simulink model "Final_Model_Building_2_AirflowAdded"  (R2022a)
settings: Solver=ode1  StartTime=0.0  StopTime=24*3600  FixedStep=10  RelTol=1e-3
values from neighbouring files (symbols this model uses):
  Aux_Threshold = 52    [Setup_Code_EWASP_VC.m]
  buildingAge = 2005    [Setup_Code_EWASP_VC.m]
  ceilingHeight = 2.4    [Setup_Code_EWASP_VC.m]
  conductiveHconnectMatrix = [ ... (first row only)    [Setup_Code_EWASP_VC.m]
  cRoofGreen = 100000    [Setup_Code_EWASP_VC.m]
  Defrost_After_Time = 30    [Setup_Code_EWASP_VC.m]
  DHWDemandProfile = occFreegainHotwaterElecTestPassiveOcc3(:,3)    [Setup_Code_EWASP_VC.m]
  Elec_Max = Elec_Max*(30/24.2)    [Setup_Code_EWASP_VC.m]
  Elec_Mid = Elec_Mid*(30/24.2)    [Setup_Code_EWASP_VC.m]
  Elec_Min = Elec_Min*(30/24.2)    [Setup_Code_EWASP_VC.m]
  ElecDemandProfile = occFreegainHotwaterElecTestPassiveOcc3(:,4)    [Setup_Code_EWASP_VC.m]
  ElecFixed = [Elec_Max(6,2) Elec_Max(6,4) Elec_Max(6,6) Elec_Max(6,7) ... (first row only)    [Setup_Code_EWASP_VC.m]
  floorOrCeilingArea = floorOrCeilingArea*1.15    [Setup_Code_EWASP_VC.m]
  forceCold = 0    [Setup_Code_EWASP_VC.m]
  freegain = occFreegainHotwaterElecTestPassiveOcc3(:,2)-max(occupancy)*25    [Setup_Code_EWASP_VC.m]
  furnitureModelOn = 1    [Setup_Code_EWASP_VC.m]
  Heat_Max = Heat_Max*(30/24.2)    [Setup_Code_EWASP_VC.m]
  Heat_Mid = Heat_Mid*(30/24.2)    [Setup_Code_EWASP_VC.m]
  Heat_Min = Heat_Min*(30/24.2)    [Setup_Code_EWASP_VC.m]
  HeatFixed = [Heat_Max(6,2) Heat_Max(6,4) Heat_Max(6,6) Heat_Max(6,7) ... (first row only)    [Setup_Code_EWASP_VC.m]
  HeatingOnProfile = repmat(HeatingOnProfile,365,1)    [Setup_Code_EWASP_VC.m]
  HEX_ReturnLowerLimit = 52.5    [Setup_Code_EWASP_VC.m]
  HEX_ReturnUpperLimit = 55    [Setup_Code_EWASP_VC.m]
  LeakMultiplier = 1+(2*(rand()-0.5)/10)    [Setup_Code_EWASP_VC.m]
  maxOcc = max(occupancyProfile)    [Setup_Code_EWASP_VC.m]
  NESW_wallArea = max(NESW_Lengths*ceilingHeight-NESW_Windows,0)    [Setup_Code_EWASP_VC.m]
  NESW_Windows = [ ... (first row only)    [Setup_Code_EWASP_VC.m]
  numRooms = roomCount    [Setup_Code_EWASP_VC.m]
  occupancy = occupancyProfile    [Setup_Code_EWASP_VC.m]
  offsetDays = 0    [Setup_Code_EWASP_VC.m]
  pumpChoice = pumpChoices(MinIndex,1)    [Setup_Code_EWASP_VC.m]
  pumpRamp = 180    [Setup_Code_EWASP_VC.m]
  ReturnLowerLimit = 37.5    [Setup_Code_EWASP_VC.m]
  ReturnUpperLimit = 40    [Setup_Code_EWASP_VC.m]
  RoofIrradiance = Flat_NS_EW_RoofIrradiance(:,1)    [Setup_Code_EWASP_VC.m]
  roofStartTemp = ones(11,1)*20    [Setup_Code_EWASP_VC.m]
  rooftype = 0    [Setup_Code_EWASP_VC.m]
  RoomDataMatrix = [zeros(1,12);ones(1,12)*wallDensity;zeros(1,12);ones(1,12)*wallU;ones(1,12)*windowU;ones(1,12)*floorU;ones(1,12)*ceilingU;zeros(1,12);windowArea, 0;floorOrCeilingArea;zeros(1,12);floorOrCeilingArea*ceilingHeight]    [Setup_Code_EWASP_VC.m]
  roomVol = roomVol*1.15    [Setup_Code_EWASP_VC.m]
  slabStartTemp = (GroundTempTimeSeries(offsetDays*1440+1,1)+thermostatSetting)/2    [Setup_Code_EWASP_VC.m]
  SlackRequest = zeros(1440,1)    [Setup_Code_EWASP_VC.m]
  SolarThermalExists = 0    [Setup_Code_EWASP_VC.m]
  SourceFixed = HeatFixed-ElecFixed    [Setup_Code_EWASP_VC.m]
  StateSeries = StateSeriesGenerator(22,7,1)    [Setup_Code_EWASP_VC.m]
  Tank_Lower_Temp = 49.5    [Setup_Code_EWASP_VC.m]
  Tank_Upper_Temp = 52    [Setup_Code_EWASP_VC.m]
  Tank_Volume_m3 = 0.15    [Setup_Code_EWASP_VC.m]
  TankHeatHour = randi([1 5])-1    [Setup_Code_EWASP_VC.m]
  upDown = [0;0;0;0;1;1;1;1;1;1;1]    [Setup_Code_EWASP_VC.m]
  wallStartTempExt = thermostatSetting*(0.266+0.00215*outdoorStartTemp+0.018*wallU+0.00113*outdoorStartTemp*wallU+0.0068*wallU^2)    [Setup_Code_EWASP_VC.m]
undefined symbols (not defined in the file or in its folder): a, ceilingU, condUDMatrix, convUDMatrix, deltaPEXPANDED_E, deltaPEXPANDED_E2, deltaPEXPANDED_N, deltaPEXPANDED_N2, deltaPEXPANDED_S, deltaPEXPANDED_S2, deltaPEXPANDED_W, deltaPEXPANDED_W2, DesiredDHWTemp, DesiredFlowTempVsInOutDeltaTemp, DiffuseHorizontal, DiscIntNeverNeededParam, DNI, dwnAndConcrete, DWORK_A_HX, DWORK_CHK_FLU, DWORK_CP_NODE, DWORK_DH, DWORK_FLUID, DWORK_HCON, DWORK_LOSS, DWORK_MDOTDOWN, DWORK_MDOTIN, DWORK_MDOTUP, DWORK_MIX, DWORK_PRESS, DWORK_QDOTIN, DWORK_RHO_NODE, DWORK_TIN, DWORK_TS_OLD, DWORK_V_NODE, ExtractRates, GroundTempTimeSeries, HCM, HCM2, HCM_closed, HCM_closed2, intermediateU, IsTop, massFlowMatrix, mechEfficiency, neighbourMatrix, numericalRoomUse, RadiatorMatrix, room2roomflowmatrix_E, room2roomflowmatrix_E2, room2roomflowmatrix_N, room2roomflowmatrix_N2, room2roomflowmatrix_S, room2roomflowmatrix_S2, room2roomflowmatrix_W, room2roomflowmatrix_W2, StateAirInEXPANDED_E, StateAirInEXPANDED_E2, StateAirInEXPANDED_N, StateAirInEXPANDED_N2 ... (+27)
libraries: simulink x6, dspsigops x4, dspmtrx3 x4, carnot x3, spsEdgeDetectorLib x2, dspstat3 x2, powerlib_meascontrol x1, simulink_extras x1
(part 6 of 27)

== system Final_Model_Building_2_AirflowAdded/GSHP_Subsystem/DHW for GSHP case ==
  note: immediately adds value to integrator to ensure legionella cycle doesnt begin right away (allows different start times)
  note: reset integrator at 00:00+delay every day,
      | so legionella cycle can start agin
  note: Makes the tank heat up to 60oC only once - only starts when the threshold programmed into switch A is hit
  note: this part prevents heating
      | to 60oC more than once per
      | day
  In1 : Inport
  In2 : Inport  Port=2
  In3 : Inport  Port=3
  In4 : Inport  Port=4
  In5 : Inport  Port=5
  In6 : Inport  Port=6
  1 means loop has been running for less than 15 mins : Switch  Criteria=u2 > Threshold  Threshold=900  SaturateOnIntegerOverflow=off  InputSameDT=off
  "1 means pump is on, and therefore ground loop is on" : Switch  Criteria=u2 > Threshold  Threshold=0.5  SaturateOnIntegerOverflow=off  InputSameDT=off
  1 means return temp recently fell below 52.1 : Relay  OnSwitchValue=61  OffSwitchValue=59  OnOutputValue=0  OffOutputValue=1  OutDataTypeStr=boolean
  1 means return temp recently fell below 52.5 : Relay  OnSwitchValue=55  OffSwitchValue=52.5  OnOutputValue=0  OffOutputValue=1  OutDataTypeStr=boolean
  1-D Lookup Table : Lookup_n-D  Commented=on  NumberOfTableDimensions=1  BreakpointsForDimension1=[0:100]  Table="[1  1\t1\t1\t1\t1\t1\t1\t1\t1\t1\t1\t1\t1\t1\t1\t1\t1\t1\t1\t1\t1\t1\t1\t1\t1\t1\t1\t1\t1\t1\t1\t1\t1\t1\t1\t1\t1\t1\t1\t1\t1\t1\t0.964285714285714\t0.931034482758621\t0.900000000000000\t0.870967741935484\t0.843750000000000\t0.818181818181818\t0.794117647058824\t0.771428571428572\t0.750000000000000\t0.729729729729730\t0.710526315789474\t0.692307692307692\t0.675000000000000\t0.658536585365854\t0.642857142857143\t0.627906976744186\t0.613636363636364\t0.600000000000000\t0.586956521739130\t0.574468085106383\t0.562500000000000\t0.551020408163265\t0.540000000000000\t0.529411764705882\t0.519230769230769\t0.509433962264151\t0.500000000000000\t0.490909090909091\t0.482142857142857\t0.473684210526316\t0.465517241379310\t0.457627118644068\t0.450000000000000\t0.442622950819672\t0.435483870967742\t0.428571428571429\t0.421875000000000\t0.415384615384615\t0.409090909090909\t0.402985074626866\t0.397058823529412\t0.391304347826087\t0.385714285714286\t0.380281690140845\t0.375000000000000\t0.369863013698630\t0.364864864864865\t0.360000000000000\t0.355263157894737\t0.350649350649351\t0.346153846153846\t0.341772151898734\t0.337500000000000\t0.333333333333333\t0.329268292682927\t0.325301204819277\t0.321428571428571\t0.317647058823529]"  InternalRulePriority=Speed  RndMeth=Simplest
  Aux Heater on1 : Logic  Inputs=3  AllPortsSameDT=off  OutDataTypeStr=boolean
  Bus Selector1 : BusSelector  OutputSignals=Pelec  OutputAsBus=on
  C/C++ Code Block : S-Function  InitFcn=try, set_param(gcb,'FunctionName','Select_sensor_mid'), end  FunctionName=Select_sensor_mid  SFunctionModules=Select_sensor_mid_wrapper  SFunctionDeploymentMode=off  EnableBusSupport=off  mask(S-Function Builder){}
      mask help: Simulink:masks:SFunctionBuilder_MD
      mask init: same as Final_Model_Building_2_AirflowAdded/ASHP_Subsystem/DHW for ASHP Case/C/C++ Code Block
      settings: CopyFcn=set_param(gcbh,'LinkStatus','none')  PreSaveFcn=try, set_param(gcb,'FunctionName','Select_sensor_mid'), end  OpenFcn=sfunctionwizard(gcbh)
      mask Display: plot(val(:,1),val(:,2)),disp(sys), port_label('input',1,'u0'), port_label('output',1,'y0')
  CHANGE to prevent 60oC being hit too often : Switch  Threshold=1  SaturateOnIntegerOverflow=off  InputSameDT=off
  Cast To Double : DataTypeConversion  OutDataTypeStr=double  SaturateOnIntegerOverflow=off  RndMeth=Floor
  Cast To Double2 : DataTypeConversion  OutDataTypeStr=double  SaturateOnIntegerOverflow=off  RndMeth=Floor
  Cast To Double3 : DataTypeConversion  OutDataTypeStr=double  SaturateOnIntegerOverflow=off  RndMeth=Floor
  Constant{1,5..6,10} (4 alike) : Constant  Value=0
  Constant11 : Constant
  Constant12 : Constant  Value=0.333
  Constant2 : Constant  Value=0.1
  Constant3 : Constant  Value=24*3600
  Constant4 : Constant
  Constant7 : Constant  Value=12
  Constant8 : Constant
  Constant9 : Constant  Value=DesiredDHWTemp
  Delay : Delay  DelayLength=1  InitialCondition=0
  Delay1 : Delay  DelayLength=1  InitialCondition=0
  Delay2 : Delay  DelayLength=1+TankHeatHour*(3600/5)  InitialCondition=0
  Delay4 : Delay  DelayLength=1  InitialCondition=0
  Digital Clock1 : DigitalClock  SampleTime=10
  Digital Clock2 : DigitalClock  SampleTime=10
  Discrete-Time Integrator : DiscreteIntegrator  ExternalReset=rising  SampleTime=-1  OutDataTypeStr=double  ICPrevOutput=DiscIntNeverNeededParam  ICPrevScaledInput=DiscIntNeverNeededParam
  Divide : Product  Inputs=*/
  Edge Detector : powerlib_meascontrol/Logic/Edge Detector  model=Rising  ic=0  Ts=-1
      settings: SourceProductBaseCode=PS
  HeatPump_Simplified : Subsystem  AncestorBlock=carnot/Source/Heat_Pump/HeatPump  mask(heat pump){Tcin=[-5 7 12], Thout=[35 45 55 60], Qdotc=[4400*a-2000*a 4200*a-2000*a 3200*a-2000*a 1800*a-2000*a;5800*a-2100*a 5500*a-2100*a 4200*a-2100*a 2800*a-2100*a;8400*a-2200*a 7200*a-2200*a 5500*a-2200*a 3300*a-2200*a], Qdoth=[4400*a 4200*a 3200*a 1800*a;5600*a 5500*a 4200*a 2800*a;8400*a 7200*a 5500*a 3300*a], Pel=[2000*a 2000*a 2000*a 2000*a;2100*a 2100*a 2100*a 2100*a;2200*a 2200*a 2200*a 2200*a], caph=10*4180, capc=4180*225, UA=7, linc=10, quac=10, linh=10, quah=10}
      mask prompts: Tcin "inlet source temperature vector (°C)"; Thout "outlet load temperature vector (°C)"; Qdotc "source power matrix (W)"; Qdoth "heating power matrix (W)"; Pel "electric power matrix (W)"; caph "thermal capacity hot loop [J/K]"; capc "thermal capacity cold loop [J/K]"; UA "heat loss coefficient [W/K]"; linc "Cold side linear massflow dependant pressure drop in [Pa*s/kg]"; quac "Cold side quadratic massflow dependant pressure drop hot side in [Pa*s²/kg]"; linh "Hot side linear massflow dependant pressure drop in [Pa*s/kg]"; quah "Hot side quadratic massflow dependant pressure drop hot side in [Pa*s²/kg]"
      mask help:
      | Linearized heat pump model. Uses measured data according to EN 14511 as input.
      | heating power: Qdot_h = K1*Tcold_in + K2*Thot_out + K3
      | electric power: Pel = K4*Tcold_in + K5*Thot_out + K6
      | source power: Qdot_c = -K7*Tcold_in - K8*Thot_out - K9
      | differential equation: cap*dTh/dt = Qdot + mdot*cp*(T_in-T) + UA*(Tamb-T)
      | with: cap = mass * heat_capactiy
      | See hp_param.m for the parameters K1 to K9.
      | Literature: Schwamberger, K.: Fortschrittsberichete VDI, Nr. 263, 1991
      mask init: same as Final_Model_Building_2_AirflowAdded/ASHP_Subsystem/DHW for ASHP Case/HeatPump_Simplified1
      mask Help: web(fullfile(path_carnot('help'),'heatpump.html'),'-helpbrowser')
      mask DialogControl ParameterTabVar0 Prompt: HP Caracteristic
      mask DialogControl ParameterTabVar01 Prompt: Thermal
      mask DialogControl ParameterTabVar012 Prompt: Hydraulic
      mask Display: plot(-20,-10,120,110,[10,20,40,60,80,90,90,80,60,40,20,10,10],[60,80,90,90,80,60,40,20,10,10,20,40,60],[40,20],[90,20],[60,80],[90,20],[50,50],[30,50],[60,40],[40,40],[57,43],[33,46],[44,57],[34,46])
  Ii : Logic  AllPortsSameDT=off  OutDataTypeStr=boolean
  Logical Operator : Logic  AllPortsSameDT=off  OutDataTypeStr=boolean
  Massflow when system is off1 : Constant  Value=0
  Max of Elements : MinMax  Function=max  Inputs=2
  Minus : Sum  Inputs=+-
  Minus1 : Sum  Inputs=+-
  Minus2 : Sum  Inputs=2
  Mod1 : Math  Operator=mod  SignedPower=on
  No DHW operation from Heat Pump : Constant  Value=0
  Plus : Sum
  Plus1 : Sum
  Product : Product
  "Run loop if either - heaing system is on, heating system was activated less than 15 mins ago" : Logic  Operator=OR  AllPortsSameDT=off  OutDataTypeStr=boolean
  S-Function Builder : S-Function  InitFcn=try, set_param(gcb,'FunctionName','Select_sensor'), end  FunctionName=Select_sensor  SFunctionModules=Select_sensor_wrapper  SFunctionDeploymentMode=off  EnableBusSupport=off  mask(S-Function Builder){}
      mask help: Simulink:masks:SFunctionBuilder_MD
      mask init: same as Final_Model_Building_2_AirflowAdded/ASHP_Subsystem/DHW for ASHP Case/C/C++ Code Block
      settings: CopyFcn=set_param(gcbh,'LinkStatus','none')  PreSaveFcn=try, set_param(gcb,'FunctionName','Select_sensor'), end  OpenFcn=sfunctionwizard(gcbh)
      mask Display: plot(val(:,1),val(:,2)),disp(sys), port_label('input',1,'u0'), port_label('output',1,'y0')
  SWITCH A : Switch  Threshold=Aux_Threshold  SaturateOnIntegerOverflow=off  InputSameDT=off
  Saturation : Saturate  UpperLimit=1  LowerLimit=0
  Scope{,1..12} (13 alike) : Scope
  Storage_Type_2_CONF : Subsystem  AncestorBlock=carnot/Storage/Thermal/Storage_Type_2_CONF  mask(Storage for hot water production){t0=52.1, hgt=1.5279, stgtype=2, tini=[52.1 52.1 52.1 52.1 52.1 52.1 52.1 52.1 52.1 52.1], mpts=[1 2 3 4 5 6 7 8 9 10], PathName=fullfile(pwd,'TankVolTemp'), FileName='<user defined>', userPath=on, userParam=on, uwall=0.235, ubot=0.235, utop=0.235, axcond=0.235, volume=Tank_Volume_m3, dia=((4/(3*3.142))*Tank_Volume_m3)^(1/3), standing=standing cylinder, nodes=10, mpoints=10, Tsensor=[0.1:0.1:0.9], hx1inlet=0.45, hx1outlet=0, hx1dia=0.03, hx1uac=500, hx1uam=0.15, hx1uat=0.6, hx1dpqua=20, hx1dplin=20, pipe1inlet=0, pipe1outlet=1, pipe1dia=0.03, pipe2inlet=0.6, pipe2outlet=1, pipe2dia=0.03}
      mask prompts: t0 "Initial temperature (vector or scalar) in °C"; hgt "Height of storage in m"; stgtype "Storage Type (0..5)"; tini "Start temperatures of nodes in °C"; mpts "Index to measured nodes"; PathName "Path"; FileName "Parameter set"; userPath "Edit path and name of parameter set"; userParam "User defined parameters"; uwall "Heat transfer coefficient to ambient [W/m²K]"; ubot "Heat transfer coefficient to ambient bottom [W/m²K]"; utop "Heat transfer coefficient to ambient top [W/m²K]"; axcond "Effective thermal conductivity [W/m/K]"; volume "Volume [m³]"; dia "Diameter [m]"; standing "Position"; nodes "Number of nodes"; mpoints "Number of node temperatures (for display)"; Tsensor "Temperature sensor position (0..1, 0 = bottom, 1 = top)"; hx1inlet "relative height of inlet"; hx1outlet "relative height of outlet"; hx1dia "Diameter of HX pipe [m]"; hx1uac "uac: heat transfer coefficient [W/K /(kg/s) /(°C)]"; hx1uam "uam: massflow dependent heat transfer [-]"; hx1uat "uat: temperature difference dependent heat transfer [-]"; hx1dpqua "pressure drop quadratic in mdot [Pa*s²/kg²]"; hx1dplin "pressure drop linear in mdot [Pa*s/kg]"; pipe1inlet "relative height of inlet, range from 0 (= bottom) to 1 (= top)"; pipe1outlet "relative height of outlet, range from 0 (= bottom) to 1 (= top)"; pipe1dia "Diameter of pipe in m"; pipe2inlet "relative height of inlet, range from 0 (= bottom) to 1 (= top)"; pipe2outlet "relative height of outlet, range from 0 (= bottom) to 1 (= top)"; pipe2dia "Diameter of pipe in m"
      mask help:
      | Storage for hot water production (domestic hot water cylinder). The storage model has the following components (with their typical position):
      | - one charging heat exchanger (lower part)
      | - one pipe connection for the hot water (total height)
      | - one pipe connection for the hot water circulation (upper part )
      mask init:
      | %[ok, param] = CarnotCallbacks_StorageConf('SetParam',stgtype,gcbh,PathName,FileName);
      mask Help: web(fullfile(path_carnot('help'),'Storage_Type_N.html'),'-helpbrowser')
      mask TypeOptions hgt: HX_EN12977_1/hgt | Pipe_Connection_1/hgt | Pipe_Connection_2/hgt
      mask TypeOptions stgtype: CreateSdat/stgtype
      mask TypeOptions tini: sfun_storageTnodesjh/tini
      mask TypeOptions mpts: select_T/Indices
      mask Callback userPath: [ok, param] = CarnotCallbacks_StorageConf('UserEdit',2,gcbh);
      mask Callback userParam: [ok, param] = CarnotCallbacks_StorageConf('UserEdit',2,gcbh);
      mask TypeOptions uwall: sfun_storageTnodesjh/uloss
      mask TypeOptions ubot: sfun_storageTnodesjh/ubot
      mask TypeOptions utop: sfun_storageTnodesjh/utop
      mask TypeOptions axcond: sfun_storageTnodesjh/cond
      mask TypeOptions volume: sfun_storageTnodesjh/volume
      mask TypeOptions dia: sfun_storageTnodesjh/dia
      mask TypeOptions standing: sfun_storageTnodesjh/standing
      mask TypeOptions nodes: sfun_storageTnodesjh/nodes | select_T/InputPortWidth | HX_EN12977_1/nodes | HX_EN12977_2/nodes | HX_EN12977_3/nodes | Pipe_Connection_1/nodes | Pipe_Connection_2/nodes | Pipe_Connection_3/nodes
      mask TypeOptions Tsensor: T_Sensor_Surface/pos
      mask TypeOptions hx1inlet: HX_EN12977_1/h_in
      mask TypeOptions hx1outlet: HX_EN12977_1/h_out
      mask TypeOptions hx1dia: HX_EN12977_1/dia
      mask TypeOptions hx1uac: HX_EN12977_1/ua0
      mask TypeOptions hx1uam: HX_EN12977_1/uam
      mask TypeOptions hx1uat: HX_EN12977_1/uat
      mask TypeOptions hx1dpqua: HX_EN12977_1/dpqua
      mask TypeOptions hx1dplin: HX_EN12977_1/dplin
      mask TypeOptions pipe1inlet: Pipe_Connection_1/h_in
      mask TypeOptions pipe1outlet: Pipe_Connection_1/h_out
      mask TypeOptions pipe1dia: Pipe_Connection_1/dia
      mask TypeOptions pipe2inlet: Pipe_Connection_2/h_in
      mask TypeOptions pipe2outlet: Pipe_Connection_2/h_out
      mask TypeOptions pipe2dia: Pipe_Connection_2/dia
      mask DialogControl Container14 Prompt: Infos
      mask DialogControl ParameterGroupVar Prompt: Picking a parameter set
      mask DialogControl Control3 Prompt: Carnot public data
      mask DialogControl Control3 Callback: [ok, file] = CarnotCallbacks_StorageConf('GetFilename',2,gcbh,'public');
      mask DialogControl Control4 Prompt: Carnot internal data
      mask DialogControl Control4 Callback: [ok, file] = CarnotCallbacks_StorageConf('GetFilename',2,gcbh,'internal');
      mask DialogControl Control2 Prompt: Selected path
      mask DialogControl Control2 Callback: [ok, file] = CarnotCallbacks_StorageConf('GetFilename',2,gcbh,'selected');
      mask DialogControl Container4 Prompt: Parameter values
      mask DialogControl Container6 Prompt: Storage
      mask DialogControl Container8 Prompt: Connections
      mask DialogControl Container11 Prompt: Heat exchanger
      mask DialogControl Container9 Prompt: Discharging pipe
      mask DialogControl Container12 Prompt: Circulation pipe
      mask DialogControl Control6 Prompt: Save in Carnot internal data
      mask DialogControl Control6 Callback: [ok, param] = CarnotCallbacks_StorageConf('SaveFilename',2,gcbh,'internal','STG');
      mask DialogControl Control5 Prompt: Save in selected path
      mask DialogControl Control5 Callback: [ok, param] = CarnotCallbacks_StorageConf('SaveFilename',2,gcbh,'selected','STG');
      mask Display:
      | % user defined picture file
      | namestr = ['Storage_Type_', num2str(get_param(gcb,'stgtype'))];
      | picfile = fullfile(path_carnot('intlibsl'), 'Storage','Thermal', ...
      |     namestr,'parameter_set', [namestr, '.jpg']);
      | 
      | % show public picture
      | plot([36,36,40,50,54,54,50,40,36]/90,...
      |     [90,50,45,45,50,90,93,93,90]/100,[36,51,44,51,36]/90,...
      |     [50,50,55,60,60]/100)
      | set_param(gcb, 'BackgroundColor', 'Red')
      | 
      | % show internal picture if defined
      | if  ~BlockIsInCarnotLibrary       % if not located in library
      |     if exist(picfile, 'file')
      |         image(imread(picfile), [0.25, 0, 0.45, 1])
      |         set_param(gcb, 'BackgroundColor', 'White')
      |     end
      | end
  Subsystem : Subsystem
      mask Display:
      | disp('Minute to \n Second Res')
      | port_label('input', 1, 'min res')
      | port_label('output', 1, 'sec res')
  Sum4 : Sum  Inputs=|++
  Switch : Switch  Criteria=u2 > Threshold  Threshold=0.1  SaturateOnIntegerOverflow=off  InputSameDT=off
  Switch Case : SwitchCase  CaseConditions={1,0}
  Switch Case Action Subsystem : Subsystem  TreatAsAtomicUnit=on
  Switch Case Action Subsystem1 : Subsystem  TreatAsAtomicUnit=on
  Switch Case Action Subsystem2 : Subsystem  TreatAsAtomicUnit=on
  Switch Case Action Subsystem3 : Subsystem  TreatAsAtomicUnit=on
  Switch Case1 : SwitchCase  CaseConditions={1,0}
  Switch1 : Switch  Criteria=u2 > Threshold  Threshold=0.5  SaturateOnIntegerOverflow=off  InputSameDT=off
  Switch5 : Switch  Criteria=u2 > Threshold  Threshold=0.5  SaturateOnIntegerOverflow=off  InputSameDT=off
  Tank Exists : Constant  Value=tankExists
  Terminator : Terminator
  Terminator1 : Terminator
  Terminator2 : Terminator
  Time since loop started flowing : Integrator  ExternalReset=rising
  over1 : Switch  Threshold=60  SaturateOnIntegerOverflow=off  InputSameDT=off
  over2 : Switch  Criteria=u2 > Threshold  SaturateOnIntegerOverflow=off  InputSameDT=off
  z{1,4,6,9} (4 alike) : Constant  Value=0
  z{2,5,7..8} (4 alike) : Constant
  Out1 : Outport  VectorParamsAs1DForOutWhenUnconnected=off
  Out2 : Outport  Port=2  VectorParamsAs1DForOutWhenUnconnected=off
  Out3 : Outport  Port=3  VectorParamsAs1DForOutWhenUnconnected=off
  Out4 : Outport  Port=4  VectorParamsAs1DForOutWhenUnconnected=off
  Out5 : Outport  Port=5  VectorParamsAs1DForOutWhenUnconnected=off
  Out6 : Outport  Port=6  VectorParamsAs1DForOutWhenUnconnected=off
  Out7 : Outport  Port=7  VectorParamsAs1DForOutWhenUnconnected=off
  Out8 : Outport  Port=8  VectorParamsAs1DForOutWhenUnconnected=off
  tag scope: AuxOn=global, NeedLegionCylce=global, WaterDemandSeries=global, loop_flow_rate=global
  wires:
  [hot_mix_fraction] -> Product/2
  Constant1/1 -> "1 means pump is on, and therefore ground loop is on"/3
  Massflow when system is off1/1 -> Switch5/3
  Switch5/1 -> Out4/1, HeatPump_Simplified/6(mdot_hot), [loop_flow_rate]
  [T_inroom] -> Storage_Type_2_CONF/1(Tamb)
  Storage_Type_2_CONF/1(Tsensors) -> S-Function Builder/1, Scope/1, C/C++ Code Block/1
  HeatPump_Simplified/1(T_source) -> Out3/1
  [DHW_on] -> "1 means pump is on, and therefore ground loop is on"/2
  Cast To Double3/1 -> Switch5/2
  [T_out] -> HeatPump_Simplified/3(Tamb)
  "1 means pump is on, and therefore ground loop is on"/1 -> HeatPump_Simplified/5(mdot_cold)
  In2/1 -> [T_inroom]
  Constant10/1 -> 1 means loop has been running for less than 15 mins/1
  [T_Source] -> HeatPump_Simplified/1(THBsource)
  Constant7/1 -> Storage_Type_2_CONF/4(THB_circ)
  Logical Operator/1 -> Cast To Double2/1
  Constant6/1 -> Storage_Type_2_CONF/6(Mdot_dhw2)
  Product/1 -> Storage_Type_2_CONF/5(Mdot_dhw1)
  Constant12/1 -> Switch5/1
  C/C++ Code Block/1 -> Out1/1, [tank_sensor_temp]
  HeatPump_Simplified/4(Real P_Therm) -> Out6/1
  1 means return temp recently fell below 52.5/1 -> Cast To Double/1
  In1/1 -> [T_Source]
  HeatPump_Simplified/3(HPdat) -> Bus Selector1/1
  Delay4/1 -> [HEX_out]
  Delay/1 -> Time since loop started flowing/1
  [DHW_on] -> Time since loop started flowing/2
  Constant11/1 -> 1 means loop has been running for less than 15 mins/3
  [DHW_on] -> "Run loop if either - heaing system is on, heating system was activated less than 15 mins ago"/1
  1 means loop has been running for less than 15 mins/1 -> "Run loop if either - heaing system is on, heating system was activated less than 15 mins ago"/2
  In5/1 -> [WaterDemandSeries]
  Time since loop started flowing/1 -> 1 means loop has been running for less than 15 mins/2
  Constant4/1 -> Delay/1
  Subsystem/1(Out1) -> Product/1
  Switch1/1 -> Out8/1, HeatPump_Simplified/4(Ctrl), [DHW_on]
  Cast To Double2/1 -> Delay1/1
  Storage_Type_2_CONF/3(THBdhw) -> Terminator2/1
  [T_mains] -> Storage_Type_2_CONF/3(THB_dhw)
  [HEX_out] -> HeatPump_Simplified/2(THB_r)
  [HEX_out] -> 1 means return temp recently fell below 52.5/1
  [WaterDemandSeries] -> Subsystem/1(In1)
  HeatPump_Simplified/2("T_out ") -> Storage_Type_2_CONF/2(Temp_HX)
  In6/1 -> "1 means pump is on, and therefore ground loop is on"/1
  [loop_flow_rate] -> Storage_Type_2_CONF/7(mdotHEX)
  In3/1 -> [T_out]
  Cast To Double/1 -> Logical Operator/1
  "Run loop if either - heaing system is on, heating system was activated less than 15 mins ago"/1 -> Ii/1
  In4/1 -> [T_mains]
  [DHW_on] -> Out2/1
  Bus Selector1/1 -> Out5/1
  Switch Case/2 -> Switch Case Action Subsystem1/Action
  Switch Case Action Subsystem1/1(Out1) -> Scope4/1, Plus/2
  [NeedLegionCylce] -> Scope9/1, Switch Case/1
  Switch Case Action Subsystem/1(Out1) -> Scope1/1, Plus/1
  [tank_sensor_temp] -> Switch Case Action Subsystem1/1(In1), Scope11/1, Switch Case Action Subsystem/1(In1)
  Switch Case/3 -> Switch Case Action Subsystem/Action
  Plus/1 -> Logical Operator/2
  Ii/1 -> Cast To Double3/1
  Switch Case Action Subsystem2/1(Out1) -> Plus1/1
  Plus1/1 -> Ii/2
  Switch Case Action Subsystem3/1(Out1) -> Plus1/2
  Switch Case1/2 -> Switch Case Action Subsystem3/Action
  [NeedLegionCylce] -> Switch Case1/1
  Switch Case1/3 -> Switch Case Action Subsystem2/Action
  [tank_sensor_temp] -> Switch Case Action Subsystem3/1(In1), Switch Case Action Subsystem2/1(In1)
  Tank Exists/1 -> Switch1/2
  No DHW operation from Heat Pump/1 -> Switch1/3
  Delay1/1 -> Switch1/1
  Storage_Type_2_CONF/4(AuxHeat) -> Out7/1
  Storage_Type_2_CONF/2(THB_hx) -> Delay4/1
  Minus2/1 -> Max of Elements/1
  Constant2/1 -> Minus2/2
  [T_mains] -> Minus1/1
  Constant9/1 -> Minus/2
  [T_mains] -> Minus/1
  Max of Elements/1 -> Minus1/2
  Minus/1 -> Divide/1
  S-Function Builder/1 -> 1-D Lookup Table/1, Max of Elements/2
  Divide/1 -> Saturation/1
  [T_mains] -> Minus2/1
  Minus1/1 -> Divide/2
  Saturation/1 -> [hot_mix_fraction]
  Aux Heater on1/1 -> Scope7/1, [AuxOn]
  Discrete-Time Integrator/1 -> [NeedLegionCylce], Scope12/1, Scope6/1, CHANGE to prevent 60oC being hit too often/2
  CHANGE to prevent 60oC being hit too often/1 -> Scope5/1, Aux Heater on1/3
  Constant8/1 -> Switch/3
  Edge Detector/1 -> Sum4/1
  over1/1 -> Scope8/1, Edge Detector/1
  Constant3/1 -> Mod1/2
  Digital Clock1/1 -> Mod1/1
  z5/1 -> SWITCH A/1
  z6/1 -> over1/3
  Sum4/1 -> Discrete-Time Integrator/1
  Delay2/1 -> Discrete-Time Integrator/2, Scope2/1
  z4/1 -> SWITCH A/3
  Constant5/1 -> Switch/1
  z8/1 -> CHANGE to prevent 60oC being hit too often/3
  z7/1 -> over1/1
  [tank_sensor_temp] -> 1 means return temp recently fell below 52.1/1, Scope10/1, over1/2, SWITCH A/2
  z2/1 -> over2/3
  1 means return temp recently fell below 52.1/1 -> Aux Heater on1/1
  over2/1 -> Sum4/2
  SWITCH A/1 -> Scope3/1, Aux Heater on1/2
  z1/1 -> over2/1
  z9/1 -> CHANGE to prevent 60oC being hit too often/1
  Mod1/1 -> Switch/2
  Digital Clock2/1 -> over2/2
  Switch/1 -> Delay2/1
  Switch Case/1 -> Terminator/1
  Switch Case1/1 -> Terminator1/1

== system Final_Model_Building_2_AirflowAdded/GSHP_Subsystem/Subsystem3 ==
  note: only required to allow me to send the
      | same signal to 2 different outputs
  note: SH GSHP
  In1 : Inport
  In2 : Inport  Port=2
  In3 : Inport  Port=3
  In4 : Inport  Port=4
  In5 : Inport  Port=5
  In6 : Inport  Port=6
  In7 : Inport  Port=7
  Bus Selector1 : BusSelector  OutputSignals=Pelec  OutputAsBus=on
  Clock4 : Clock
  Data Type Conversion2 : DataTypeConversion  OutDataTypeStr=double  SaturateOnIntegerOverflow=off  RndMeth=Floor
  Data Type Conversion3 : DataTypeConversion  OutDataTypeStr=double  SaturateOnIntegerOverflow=off  RndMeth=Floor
  Data Type Conversion4 : DataTypeConversion  OutDataTypeStr=double  SaturateOnIntegerOverflow=off  RndMeth=Floor
  Ground_Source_Heat_Exchanger1 : Subsystem  AncestorBlock=carnot/Source/Heat_Pump/Ground_Source_Heat_Exchanger  mask(vertical ground source heat exchanger){Jahresmitteltemp_C=12, TGrad=0.025, lambdaErde=5, cpErde=11000, rhoErde=2500, lambdaFill=5, cpFill=1000, rhoFill=2000, Sondelaenge=100, B=10, Sondendurchmesser=0.032, Bohrdurchmesser=0.18, sondenfall=2 probes B/H = 0.1, np=2, DimAxi=10, DimRad=10, Gitterfaktor=2.5}
      mask prompts: Jahresmitteltemp_C "Average annual outdoor temperature  in °C"; TGrad "Temperature gradient in K/m, typical 0.025..0.04"; lambdaErde "Thermal conductivity ground in W/m/K"; cpErde "Heat capacity of the ground in J/kg/K"; rhoErde "Denstiy of the ground in kg/m³"; lambdaFill "Thermal conductivity filling in W/m/K"; cpFill "Heat capacity of the filling in J/kg/K"; rhoFill "Denstiy of the filling in kg/m³"; Sondelaenge "H: Length of earth probe in m"; B "B: probe distance in m"; Sondendurchmesser "Diameter of tube in m"; Bohrdurchmesser "Diameter of drilled hole in m"; sondenfall "Field geometry"; np "Number of parallel tubes"; DimAxi "No. of nodes in axial direction (typical 10)"; DimRad "No. of nodes in radial direction (typical 10)"; Gitterfaktor "grid factor (typical 2.5)"
      mask help:
      | The CARNOT EWS model is a transient model for dynamic simulation of borehole heat exchangers or so-called vertical ground heat exchangers. The model is based on the equations described by [Huber97] and has been implemented using the state space model of Matlab/Simulink [Bianchi06].
      | Bianchi M. A., Adaptive modellbasierte prädiktive Regelung einer Kleinwärmepumenanlage Diss. ETH Zuerich, No. 16892, 2006
      | Huber A, Schuler O., Berechnungsmodul für Erdwärmesonden (EWS). ENET Bericht Nr. 9658807-1, 1997
      mask init:
      | % Sets the parameters for the model
      | % ***********************************************************************
      | % This file is part of the CARNOT Blockset.
      | %   CARNOT is free software: you can redistribute it and/or modify
      | %   it under the terms of the GNU Lesser General Public License as published by
      | %   the Free Software Foundation, either version 3 of the License, or
      | %   (at your option) any later version.
      | %   CARNOT is distributed in the hope that it will be useful,
      | %   but WITHOUT ANY WARRANTY; without even the implied warranty of
      | %   MERCHANTABILITY or FITNESS FOR A PARTICULAR PURPOSE.  See the
      | %   GNU Lesser General Public License for more details.
      | %   You should have received a copy (copying_lesser.txt) of the 
      | %   GNU Lesser General Public License along with CARNOT.  
      | %   If not, see <http://www.gnu.org/licenses/>.
      | %  
      | % **********************************************************************
      | % author list:      fab -> Fabian Ochs
      | %                   hf  -> Bernd Hafner
      | %
      | % version: CarnotVersion.MajorVersionOfFunction.SubversionOfFunction
      | %
      | % Version  Author  Changes                                     Date
      | % 5.1.0    fab     created, based on Diss. Bianchi ETH Zurich  01dec2012
      | % 5.1.1    hf      adapted to carnot input and output struct.  04mar2013 
      | %
      | % Copyright (c) 2012 TU Insbruck, Fabian Ochs
      | 
      | startfall = 2; % 2: g-function
      | mdot = 0.5;
      | teta_in = 1;
      | Massenstrom = mdot/np;
      | Qdot0 = 5000;
      | t_start = 50*8560*3600;
      | 
      | % Geometry
      | Dicke_Sondenrohr = 0.003;
      | lambda_Sondenrohr = 0.48;
      | Bu = .1293;
      | 
      | % Ground Properties
      | aErde = lambdaErde/(rhoErde*cpErde);
      | 
      | % Fluid
      | teta_m = 2; 
      | p0 = 1E5;
      | fluid = 5;
      | mix = 0.25;
      | 
      | Jahresmitteltemp=Jahresmitteltemp_C + 273.15;
      | Bodenerwaermung=1;                          % 0°C
      | Bodentemp=Jahresmitteltemp+Bodenerwaermung; % K
      | 
      | % Calculation
      | lambdaSole=thermal_conductivity(teta_m,p0,fluid,mix);%W/(m K)
      | cpSole=heat_capacity(teta_m,p0,fluid,mix);                                % J/Kg*K
      | rhoSole=density(teta_m,p0,fluid,mix);%kg/m^3
      | vSole=kinematic_viscosity(teta_m,p0,fluid,mix);                             % m2/s
      | 
      | Pr=vSole*rhoSole*cpSole/lambdaSole;
      | rb = Bohrdurchmesser/2;
      | rm = B/2;
      | Rechenradius = rm;
      | Dl=Sondelaenge/DimAxi*2;    
      | 
      | rs=Sondendurchmesser/2;
      | r0 = rs-Dicke_Sondenrohr; % Innenradius
      | r1=Bohrdurchmesser/2;
      | r2=r1+(Rechenradius-r1)*(1-Gitterfaktor)/(1-Gitterfaktor^(DimRad-1))*Gitterfaktor^0;
      | 
      | rz1=((r1^2+r0^2)/2)^0.5;
      | rz2=((r2^2+r1^2)/2)^0.5;
      | 
      | mcpSole=2*cpSole*rhoSole*pi*Dl*(Sondendurchmesser/2)^2;
      | Di = Sondendurchmesser - 2 * Dicke_Sondenrohr;
      | Geschw_Sole= Massenstrom/rhoSole/(Di/2)^2/pi/2; % 2: double U
      | 
      | Vdot = Massenstrom/rhoSole;
      | A_p = (Di/2)^2/pi/2;
      | 
      | Re=Geschw_Sole*Di/vSole;
      | Druckverlust= 1/(1.82*log10(Re)-1.64)^2;
      | K1=1+27.2*Druckverlust/8;
      | K1_o=1.106886;
      | K2=11.7+1.8*Pr^(-1.3);
      | Druckverlust_o=0.031437;
      | St_o= Druckverlust_o/8/(K1_o+K2*(Druckverlust_o/8)^0.5*(Pr^(2/3)-1));
      | Nu_o=St_o*10000*Pr;
      | St= Druckverlust/8/(K1+K2*(Druckverlust/8)^0.5*(Pr^(2/3)-1));
      | 
      | % acc. Hellström    
      | b = Bu/(2*r1);
      | b_max = 1-rs/r1;
      | b_min = rs/r1;
      | sigma = (lambdaFill-lambdaErde)/(lambdaErde+lambdaFill);
      | A = pi*r0^2;
      | vs = Massenstrom/2/rhoSole/A;
      | zeta = 1/((1.82*log10(Re)-1.64)^2);
      | K1 = 1+27.2*zeta/8;
      | K2 = 11.7+1.8*Pr^(-1/3); 
      | R_s = 1/(2*pi*lambda_Sondenrohr)*log(rs/r0);
      |     
      | Nu_turbulent=St*Re*Pr;        
      | Nu_laminar=4.36;
      | 
      | if Re>=10000,
      |     Nu =(zeta/8)*Re*Pr/(K1+K2*(zeta/8)^.5*(Pr^(2/3)-1));
      | elseif Re<10000 && Re>2300
      |     Nu = Nu_laminar*exp(log(Nu_o/Nu_laminar)*log(Re/2300)/log(10000/2300));
      | elseif Re<=2300,
      |     Nu=Nu_laminar;        
      | end
      |     
      | alpha = Nu*lambdaSole/(2*r0);
      | alpha_eff = (1/alpha+r0/lambda_Sondenrohr*log(rs/r0))^-1;
      | alpha0 = lambdaSole/(Di/2*(1-0.5^0.5));
      | alpha0_eff = (1/alpha0+r0/lambda_Sondenrohr*log(rs/r0))^-1;
      | 
      | R_a = 1/(8*pi*alpha*r0);
      | beta = lambdaFill*(1/(r0*alpha)+1/lambda_Sondenrohr*log(rs/r0));
      | 
      | R1_EWS=0.25*(1/(2*pi*alpha_eff*r0*Dl)+1/(2*pi*lambdaFill*Dl)*log((r1-rz1)/r0));
      | R2_EWS=1/(2*pi*Dl)*(1/lambdaFill*log(r1/rz1)+1/lambdaErde*log(rz2/r1));        
      | R10_EWS=0.25*(1/(2*pi*alpha0_eff*r0*Dl)+1/(2*pi*lambdaFill*Dl)*log((r1-rz1)/r0));
      | R20_EWS=1/(2*pi*Dl)*(1/lambdaFill*log(r1/rz1)+1/lambdaErde*log(rz2/r1));        
      | 
      | Ra = 1/(pi*lambdaFill)*(log((2^.5*b*r1)/r0)-1/2*log((2*b*r1)/r0)-1/2*sigma*log((1-b^4)/(1+b^4)))+(1/(2*pi*r0*alpha))+R_s;
      | Rb = (1/(8*pi*lambdaFill))*(beta+log(r1/r0)+log(r1/Bu)+sigma*log(r1^4/(r1^4-Bu^4/16))-(r0^2/Bu^2*(1-sigma*(Bu^474)/(r1^4-Bu^4/16)^2))/((1+beta)/(1-beta)+r0^2/Bu^2*(1+sigma*Bu^4*r1^4/(r1^4-Bu^4/16)^2)));
      | Ra0 = 1/(pi*lambdaFill)*(log((2^.5*b*r1)/r0)-1/2*log((2*b*r1)/r0)-1/2*sigma*log((1-b^4)/(1+b^4)))+(1/(2*pi*r0*alpha0))+R_s;
      | Rb0 = (1/(8*pi*lambdaFill))*(beta+log(r1/r0)+log(r1/Bu)+sigma*log(r1^4/(r1^4-Bu^4/16))-(r0^2/Bu^2*(1-sigma*(Bu^474)/(r1^4-Bu^4/16)^2))/((1+beta)/(1-beta)+r0^2/Bu^2*(1+sigma*Bu^4*r1^4/(r1^4-Bu^4/16)^2)));
      | 
      | if Ra < 4 * Rb
      |     R1 = Ra/(4*Dl);
      |     R2 = (Rb-Ra/4)/Dl+(2*pi*Dl*lambdaErde)^-1*log(rz2/r1);
      |     R10 = Ra0/(4*Dl);
      |     R20 = (Rb0-Ra0/4)/Dl+(2*pi*Dl*lambdaErde)^-1*log(rz2/r1);        
      | else
      |     R1 = R1_EWS;
      |     R2 = R2_EWS;
      |     R10 = R10_EWS;
      |     R20 = R20_EWS;
      | end
      |     
      | % temperaturverlauf axialer richtung
      | L0=cpSole*Massenstrom;      % konstant
      | L00 = 0.0;
      | L1=1/R1;
      | L2=1/R2;
      | L10=1/R10;
      | L20=1/R20;
      | 
      | % matrizen Ad,Bd,Cd,Dd für Tdown
      | Ad=zeros(DimAxi/2,DimAxi/2);
      | Ad0=zeros(DimAxi/2,DimAxi/2);
      | for h=1:DimAxi/2,
      |     Ad(h,h)=-(L0/(mcpSole)+L1/(2*mcpSole));
      |     Ad0(h,h)=-(L00/(mcpSole)+L10/(2*mcpSole));
      | end
      |   
      | for h=1:DimAxi/2-1,
      |     Ad(h+1,h)=L0/(mcpSole);
      |     Ad0(h+1,h)=L00/(mcpSole);
      | end
      | 
      | Bd=zeros(DimAxi/2,DimAxi/2+1);
      | Bd0=zeros(DimAxi/2,DimAxi/2+1);
      | Bd(1,1)=L0/(mcpSole);
      | Bd0(1,1)=L00/(mcpSole);
      | 
      | for h=1:DimAxi/2,
      |     Bd(h,h+1)=L1/(2*mcpSole);
      |     Bd0(h,h+1)=L10/(2*mcpSole);
      | end
      | 
      | Cd=eye(DimAxi/2);
      | Dd=zeros(DimAxi/2,DimAxi/2+1);
      | 
      | % matrizen Au,Bu,Cu,Du für Tup
      | Au=zeros(DimAxi/2,DimAxi/2);
      | Au0=zeros(DimAxi/2,DimAxi/2);
      | for h=1:DimAxi/2,
      |     Au(h,h)=-(L0/(mcpSole)+L1/(2*mcpSole));
      |     Au0(h,h)=-(L00/(mcpSole)+L10/(2*mcpSole));
      | end
      |   
      | for h=1:DimAxi/2-1,
      |     Au(h+1,h)=L0/(mcpSole);
      |     Au0(h+1,h)=L00/(mcpSole);
      | end
      | 
      | Bu=zeros(DimAxi/2,DimAxi/2+1);
      | Bu0=zeros(DimAxi/2,DimAxi/2+1);
      | Bu(1,1)=L0/(mcpSole);
      | Bu0(1,1)=L00/(mcpSole);
      | for h=1:DimAxi/2,
      |     Bu(h,h+1)=L1/(2*mcpSole);
      |     Bu0(h,h+1)=L10/(2*mcpSole);
      | end
      | 
      | Cu=Cd;
      | Du=zeros(DimAxi/2,DimAxi/2+1);
      | 
      | % berechnung von Tradial, von Luzi Valär
      | Dim1=(DimRad-2)*DimAxi/2;
      | r = zeros(1:DimRad);
      | r(1)=Bohrdurchmesser/2;
      | r(2)=r2;
      | for h =3:DimRad,
      |     r(h)=r(h-1)+(Rechenradius-r1)*(1-Gitterfaktor)/(1-Gitterfaktor^(DimRad-1))*Gitterfaktor^(h-2);
      | end
      |     
      | rz = zeros(1:DimRad);
      | rz(1)=((r(1)^2+r0^2)/2)^0.5;
      | for h = 2:DimRad,
      |     rz(h)=((r(h)^2+r(h-1)^2)/2)^0.5;
      | end
      | 
      | L = zeros(1:DimRad);
      | L(1)=L1; 
      | L(2)=L2;
      | for h = 3:DimRad-1,
      |     L(h)=1/(1/(2*pi*Dl)*(1/lambdaErde*log(rz(h)/rz(h-1))));
      | end
      | L(DimRad)=1/(1/(2*pi*Dl)*(1/lambdaErde*log(r(DimRad)/rz(DimRad-1))));
      | 
      | 
      | C = zeros(1:DimRad);
      | C(1)=cpFill*rhoFill*pi*(r(1)^2-4*r0^2)*Dl;
      | for h = 2:DimRad,
      |     C(h)=cpErde*rhoErde*pi*(r(h)^2-r(h-1)^2)*Dl;
      | end
      | 
      | 
      | a=zeros(DimRad-2,DimRad-2);
      | for h = 1:DimRad-2,
      |     a(h,h)=(-L(h)-L(h+1))/C(h);
      | end
      | for h = 1:DimRad-3,
      |     a(h,h+1)=L(h+1)/C(h);
      |     a(h+1,h)=L(h+1)/C(h+1);
      | end
      | 
      | b=zeros(DimRad-2,2);
      |     b(1,1)=L(1)/C(1);
      |     b(DimRad-2,2)=L(DimRad-1)/C(DimRad-2);
      |     
      | %%%%%%%%%%%%%%%%%%%%%%%%%%%%%%%%%%%%%%%%%%%%%%%%%%% 
      |     
      | Ar=a;
      | Ar(DimRad-1:2*(DimRad-2),DimRad-1:2*(DimRad-2))=a;
      |     
      | for h=2:DimAxi/2-1,
      |     Ar(h*(DimRad-2)+1:(h+1)*(DimRad-2),h*(DimRad-2)+1:(h+1)*(DimRad-2))=a;
      | 
      | end  
      | 
      | Br=b;
      | 
      | for h=1:DimAxi/2-1,
      |     Br(h*(DimRad-2)+1:(h+1)*(DimRad-2),2*h+1:2*h+2)=b;   
      | end
      |     
      | 
      | Cr=eye((DimRad-2)*DimAxi/2);
      | Dr=zeros((DimRad-2)*DimAxi/2,DimAxi);
      | 
      | % andere matrizen
      | Cdl=zeros(DimAxi/2,1);
      | Cdl(DimAxi/2,1)=1;
      | Cdl=Cdl';
      | 
      | c1=zeros(DimAxi/2,Dim1);
      | for h=1:DimAxi/2,
      |     c1(1,1)=1;
      |     c1(h,(h-1)*(DimRad-2)+1)=1;
      | end
      | 
      | c31=zeros(1,DimAxi/2);
      | c3(1,1)=1;
      | for h=1:DimAxi/2-1,
      |     c3(1+2*h,1+h)=1;
      | end
      | 
      | c33=zeros(DimAxi,DimAxi/2);
      | c33(1:DimAxi-1,1:DimAxi/2)=c3;
      | 
      | c41=zeros(1,DimAxi/2);
      | c4=c41;
      | c4(2:DimAxi,1:DimAxi/2)=c3;
      | 
      | 
      | % randbedingungen für Tearth,DimRad
      | % anfangsbedingungen für Tradial
      | mu=linspace(0,Sondelaenge,DimAxi/2);
      | T=(mu*TGrad+Bodentemp);
      | Tearth_anf=T'*ones(1,DimRad-2);
      | T_null=Tearth_anf(:,1);
      | teta_fluid_ini = mean(T_null)-273.15;
      | 
      | % anfangsbedingungen für Tdown,Tup
      | Tdown_0=Tearth_anf(:,1);
      | Tup_0=flipud(Tdown_0);
      | Tearth_anf=Tearth_anf';
      | c5=ones(DimAxi/2,1);           
      | 
      | c6=zeros(DimRad-2,3*(DimRad-2));
      | 
      | for i=2:DimRad-2;
      |     c6(1,DimRad-1)=1;
      |     c6(i,DimRad+i-2)=1;
      | end
      | 
      | %% RB
      | Ts_Trichter=7*24*3600; % 7 (1 week according to Huber)
      | Dr_Trichter=1;
      | t_Trichter = linspace(Ts_Trichter,Ts_Trichter*5000,5000);
      | r_Trichter = linspace(Dr_Trichter,Dr_Trichter*20,20);
      | 
      | % g-function
      | xS = [-4 -2 0 2 3];
      | if sondenfall == 1          % 1 Sonde
      |     yS = [4.82 5.69 6.29 6.57 6.6];
      | elseif sondenfall == 2      % 2 Sonden B/H = 0.1
      |     yS = [4.99 6.37 7.62 8.06 8.08];
      | elseif sondenfall == 3      % 2 Sonden B/H = 0.05
      |     yS = [5.30 6.92 8.20 8.67 8.71];
      | elseif sondenfall == 4      % 3x6 Sonden B/H = 0.1
      |     yS = [5.00 9.15 16.40 19.75 20.05];
      | elseif sondenfall == 5      % 5x10 Sonden B/H = 0.1
      |     yS = [5.00 10.2 22.75 29.5 30.05];
      | end
      | 
      | npol = 4;
      | p = polyfit(xS,yS,npol);
      | ts = Sondelaenge^2/(9*aErde);
      | gfunction = zeros(length(t_Trichter),length(r_Trichter));
      | Es = t_Trichter*9*aErde/Sondelaenge^2;
      | 
      | g = polyval(p,log(Es));
      | 
      | for ii = 1:length(r_Trichter)
      |     gfunction(:,ii) = max(0,g - log(r_Trichter(ii)/Sondelaenge/0.0005)); % correction 21-09-2012
      | end
      | 
      | % Startwerte
      | qdot0 = Qdot0/Sondelaenge; 
      | if startfall == 2
      |     Es_start = t_start*9*aErde/Sondelaenge^2;
      |     TEarth0 = zeros(size(Tearth_anf));
      |     for ii = 1:DimAxi/2
      |         for iii = 1:DimRad-1
      |             g_start = polyval(p,log(Es_start));
      |             TEarth0(iii,ii) = Bodentemp + mu(ii)*TGrad - qdot0/(DimAxi/2)*((g_start-log(rz(iii+1)/Sondelaenge/0.0005))/(2*pi*lambdaErde));
      |         end
      |     end    
      | 
      |     T_null = TEarth0(end,:)';
      |     Tearth_anf = TEarth0(1:end-1,:);
      | end
      mask Help: web(['file:///' fullfile(path_carnot('help'),'Ground_Source_Heat_Exchanger.html')],'-helpbrowser')
      mask TypeOptions sondenfall: 1 probe | 2 probes B/H = 0.1 | 2 probes B/H = 0.05 | 3x6 probes B/H = 0.1 | 5x10 probes B/H = 0.1
      mask DialogControl ParameterTabVar0 Prompt: General
      mask DialogControl ParameterTabVar01 Prompt: Geometry
      mask DialogControl ParameterTabVar012 Prompt: Calculation
      mask Display:
      | plot(0,10,100,90,[70,30],[80,80],[35,35,43,43,47,52,57,57,66,66,60,60,54,46,40,40,35],[84,87,87,20,13,13,21,87,87,84,84,20,10,10,20,84,84])
      | port_label('input',1,'Tin')
      | port_label('input',2,'Mdot')
      | port_label('output',1,'THB')
      | port_label('output',2,'Tn')
  HeatPump_Simplified : Subsystem  AncestorBlock=carnot/Source/Heat_Pump/HeatPump  mask(heat pump){Tcin=[-5 7 12], Thout=[35 45 55 60], Qdotc=[4400*a-2000*a 4200*a-2000*a 3200*a-2000*a 1800*a-2000*a;5800*a-2100*a 5500*a-2100*a 4200*a-2100*a 2800*a-2100*a;8400*a-2200*a 7200*a-2200*a 5500*a-2200*a 3300*a-2200*a], Qdoth=[4400*a 4200*a 3200*a 1800*a;5600*a 5500*a 4200*a 2800*a;8400*a 7200*a 5500*a 3300*a], Pel=[2000*a 2000*a 2000*a 2000*a;2100*a 2100*a 2100*a 2100*a;2200*a 2200*a 2200*a 2200*a], caph=10*4180, capc=4180*225, UA=2, linc=10, quac=10, linh=10, quah=10}
      mask prompts: Tcin "inlet source temperature vector (°C)"; Thout "outlet load temperature vector (°C)"; Qdotc "source power matrix (W)"; Qdoth "heating power matrix (W)"; Pel "electric power matrix (W)"; caph "thermal capacity hot loop [J/K]"; capc "thermal capacity cold loop [J/K]"; UA "heat loss coefficient [W/K]"; linc "Cold side linear massflow dependant pressure drop in [Pa*s/kg]"; quac "Cold side quadratic massflow dependant pressure drop hot side in [Pa*s²/kg]"; linh "Hot side linear massflow dependant pressure drop in [Pa*s/kg]"; quah "Hot side quadratic massflow dependant pressure drop hot side in [Pa*s²/kg]"
      mask help:
      | Linearized heat pump model. Uses measured data according to EN 14511 as input.
      | heating power: Qdot_h = K1*Tcold_in + K2*Thot_out + K3
      | electric power: Pel = K4*Tcold_in + K5*Thot_out + K6
      | source power: Qdot_c = -K7*Tcold_in - K8*Thot_out - K9
      | differential equation: cap*dTh/dt = Qdot + mdot*cp*(T_in-T) + UA*(Tamb-T)
      | with: cap = mass * heat_capactiy
      | See hp_param.m for the parameters K1 to K9.
      | Literature: Schwamberger, K.: Fortschrittsberichete VDI, Nr. 263, 1991
      mask init: same as Final_Model_Building_2_AirflowAdded/ASHP_Subsystem/DHW for ASHP Case/HeatPump_Simplified1
      mask Help: web(fullfile(path_carnot('help'),'heatpump.html'),'-helpbrowser')
      mask DialogControl ParameterTabVar0 Prompt: HP Caracteristic
      mask DialogControl ParameterTabVar01 Prompt: Thermal
      mask DialogControl ParameterTabVar012 Prompt: Hydraulic
      mask Display: plot(-20,-10,120,110,[10,20,40,60,80,90,90,80,60,40,20,10,10],[60,80,90,90,80,60,40,20,10,10,20,40,60],[40,20],[90,20],[60,80],[90,20],[50,50],[30,50],[60,40],[40,40],[57,43],[33,46],[44,57],[34,46])
  Instantaneous to kWh Total2 : Subsystem
  Logical Operator : Logic  Operator=NOT  AllPortsSameDT=off  OutDataTypeStr=boolean
  Logical Operator1 : Logic  AllPortsSameDT=off  OutDataTypeStr=boolean
  Logical Operator2 : Logic  Operator=NOT  AllPortsSameDT=off  OutDataTypeStr=boolean
  Logical Operator3 : Logic  Operator=OR  AllPortsSameDT=off  OutDataTypeStr=boolean
  Logical Operator6 : Logic  Inputs=3  AllPortsSameDT=off  OutDataTypeStr=boolean
  Massflow when system is off : Constant  Value=0
  Massflow when system is off1 : Constant  Value=0
  Massflow when system is on : Constant  Value=3400/3600
  Plus : Sum
  Relay2 : Relay  OnSwitchValue=ReturnUpperLimit  OffSwitchValue=ReturnLowerLimit  OnOutputValue=0  OffOutputValue=1  OutDataTypeStr=boolean
  Scope3 : Scope
  Switch1 : Switch  Criteria=u2 > Threshold  Threshold=0.5  SaturateOnIntegerOverflow=off  InputSameDT=off
  Switch5 : Switch  Criteria=u2 > Threshold  Threshold=0.5  SaturateOnIntegerOverflow=off  InputSameDT=off
  Switch6 : Switch  Criteria=u2 > Threshold  Threshold=10  SaturateOnIntegerOverflow=off  InputSameDT=off
  Terminator8 : Terminator
  on? (I/O)9 : Constant  Value=20  OutDataTypeStr=double
  tank_sensor_temp4 : Scope
  tank_sensor_temp5 : Scope
  x : Constant  Value=0
  Out1 : Outport  VectorParamsAs1DForOutWhenUnconnected=off
  Out2 : Outport  Port=2  VectorParamsAs1DForOutWhenUnconnected=off
  Out3 : Outport  Port=3  VectorParamsAs1DForOutWhenUnconnected=off
  Out4 : Outport  Port=4  VectorParamsAs1DForOutWhenUnconnected=off
  Out5 : Outport  Port=5  VectorParamsAs1DForOutWhenUnconnected=off
  Out6 : Outport  Port=6  VectorParamsAs1DForOutWhenUnconnected=off
  Out7 : Outport  Port=7  VectorParamsAs1DForOutWhenUnconnected=off
  Out8 : Outport  Port=8  VectorParamsAs1DForOutWhenUnconnected=off
  wires:
  In2/1 -> [MixedTemp]
  [pump_power_Fraction] -> HeatPump_Simplified/7(power fraction)
  Switch6/1 -> Relay2/1, HeatPump_Simplified/2(THB_r)
  Logical Operator/1 -> Logical Operator6/3
  x/1 -> Plus/2
  Relay2/1 -> Logical Operator6/1
  Massflow when system is on/1 -> Switch1/1
  Ground_Source_Heat_Exchanger1/2(Tnodes) -> tank_sensor_temp4/1, Terminator8/1
  HeatPump_Simplified/4(Real P_Therm) -> Out4/1, Instantaneous to kWh Total2/1(In1)
  Ground_Source_Heat_Exchanger1/1(Tout) -> Out8/1, [FromGround]
  [T_Out] -> HeatPump_Simplified/3(Tamb)
  [Global_Control_Signal] -> Logical Operator1/1
  Data Type Conversion2/1 -> Out1/1, Plus/1, HeatPump_Simplified/4(Ctrl)
  HeatPump_Simplified/1(T_source) -> Out6/1
  Bus Selector1/1 -> Out5/1
  In3/1 -> [MassFlowTotal]
  Clock4/1 -> Switch6/2
  Switch5/1 -> HeatPump_Simplified/6(mdot_hot), Out7/1, tank_sensor_temp5/1
  on? (I/O)9/1 -> Switch6/3
  HeatPump_Simplified/2("T_out ") -> Out3/1
  [DHW_on] -> Logical Operator3/2
  [Global_Control_Signal] -> Logical Operator6/2
  [Global_Control_Signal] -> Logical Operator3/1
  Switch1/1 -> [mdot_cold], Ground_Source_Heat_Exchanger1/2(Mdotin1)
  In1/1 -> [T_Out]
  Logical Operator3/1 -> Data Type Conversion4/1
  Massflow when system is off1/1 -> Switch5/3
  HeatPump_Simplified/3(HPdat) -> Bus Selector1/1
  [ToGroundTot] -> Ground_Source_Heat_Exchanger1/1(Tin)
  In4/1 -> [Global_Control_Signal]
  Data Type Conversion4/1 -> Switch1/2
  Logical Operator2/1 -> Logical Operator1/2
  [DHW_on] -> Logical Operator/1
  [MixedTemp] -> Switch6/1
  Massflow when system is off/1 -> Switch1/3
  Logical Operator6/1 -> Data Type Conversion2/1
  [MassFlowTotal] -> Switch5/1
  [mdot_cold] -> HeatPump_Simplified/5(mdot_cold)
  Instantaneous to kWh Total2/1(Out1) -> Scope3/1
  Logical Operator1/1 -> Data Type Conversion3/1
  In5/1 -> [pump_power_Fraction]
  [FromGround] -> HeatPump_Simplified/1(THBsource)
  Data Type Conversion3/1 -> Switch5/2
  In6/1 -> Logical Operator2/1
  In7/1 -> [ToGroundTot]
  Plus/1 -> Out2/1
